simulink model "am_mod"  (R2023b)
settings: Solver=VariableStepAuto  StartTime=0.0  StopTime=0.1  RelTol=1e-3
values from neighbouring files (symbols this model uses):
  fc_mod_fm = 110e3    (= 110000)    [simulink_parametros.m]
  fc_test_mod_am = 10*fm_test_mod_am    (= 10000)    [simulink_parametros.m]
  fm_test_mod_am = 1000    [simulink_parametros.m]
  ts_test_mod_am = 1/fs_test_mod_am    (= 1e-05)    [simulink_parametros.m]
undefined symbols (not defined in the file or in its folder): BE, ode23tb, trap
libraries: rfmathmodels2 x1
settings Model: Creator=RomaW11  LastModifiedBy=RomaW11

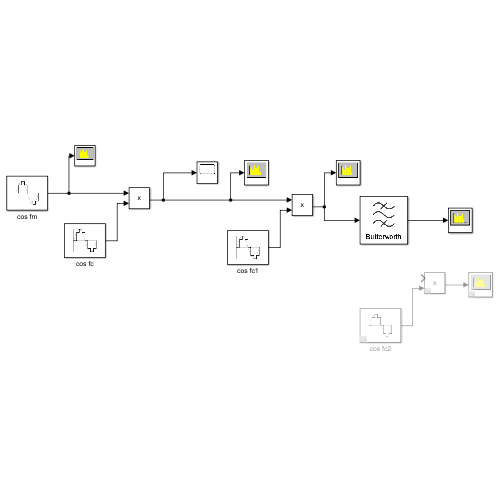
[thumbnail: Simulink's stored preview of the top-level diagram]
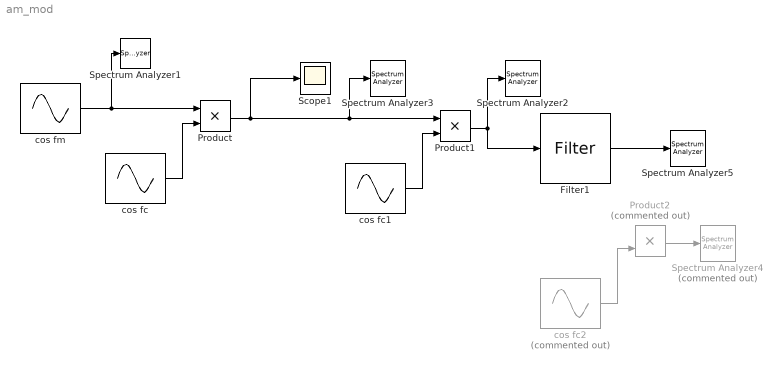
== system am_mod ==
  Filter1 : rfmathmodels2/Filter  DesignMethod=Butterworth  ResponseType=Bandpass  UseFilterOrder=on  FilterOrder=3  PassFreq_lp=1e9  PassFreq_hp=2000000000  PassFreq_bp=[15e3 25e3]  PassFreq_bs=[1000000000 4000000000]  PassAtten=10*log10(2)  StopFreq_lp=2000000000  StopFreq_hp=1000000000  StopFreq_bp=[1500000000 3500000000]  StopFreq_bs=[2100000000 2900000000]  StopAtten=40  CarrierFrequency=20e3  SignalBandwidth=10000000  SimulateUsing=Interpreted execution  ModelingDomain=Time domain (Fixed step)  SolverFixedStep=NDF2  SolverODE=ode23tb (trap+BE)  PoleFitting=Share all poles  RationalArguments={ 'Tolerance', -40, 'TendsToZero', false, 'MaxPoles', 48, 'Qlimit', inf }  LengthFIR=128  PlotType1=S21  Plot1Units=Magnitude (dB)  Plot1ArgumentsImpulse=[1e-11 1e4]  Plot1ArgumentsStep=[1e-11 1e4 1e-10]  PlotType2=None  Plot2Units=Magnitude (dB)  Plot2ArgumentsImpulse=[1e-11 1e4]  Plot2ArgumentsStep=[1e-11 1e4 1e-10]  FrequencyPoints=logspace(8,10,2001)  XaxisScale=Linear  YaxisScale=Linear
  Product : Product
  Product1 : Product
  Product2 : Product  Commented=on
  Scope1 : Scope
  Spectrum Analyzer1 : SpectrumAnalyzer  WindowPosition=[7.000000,-1079.000000,1920.000000,1057.000000,]  ScopeFrameLocation=window  SampleRate=44.1e3  StartFrequency=20  StopFrequency=20e3  YLimits=[-53.06122828,27.41733441]
      settings: OpenAtSimulationStart=off
  Spectrum Analyzer2 : SpectrumAnalyzer  WindowPosition=[7.000000,-1079.000000,1920.000000,1057.000000,]  ScopeFrameLocation=window  SampleRate=44.1e3  StartFrequency=20  StopFrequency=20e3  YLimits=[-52.30886083,20.64603656]  SelectedToolstripTab=spectrumAnalyzerToolstrip.estimationTab
      settings: OpenAtSimulationStart=off
  Spectrum Analyzer3 : SpectrumAnalyzer  WindowPosition=[1.000000,1.000000,1920.000000,1057.000000,]  ScopeFrameLocation=window  SampleRate=44.1e3  StartFrequency=20  StopFrequency=20e3  YLimits=[-52.32816931,20.81980716]
      settings: OpenAtSimulationStart=off
  Spectrum Analyzer4 : SpectrumAnalyzer  Commented=on  WindowPosition=[1.000000,1.000000,1920.000000,1057.000000,]  ScopeFrameLocation=window  SampleRate=44.1e3  StartFrequency=20  StopFrequency=20e3  YLimits=[-51.57709306,14.06031154]  SelectedToolstripTab=spectrumAnalyzerToolstrip.estimationTab
      settings: OpenAtSimulationStart=off
  Spectrum Analyzer5 : SpectrumAnalyzer  WindowPosition=[7.000000,-1079.000000,1920.000000,1057.000000,]  ScopeFrameLocation=window  SampleRate=44.1e3  StartFrequency=20  StopFrequency=20e3  YLimits=[-51.57709306,14.06031154]  SelectedToolstripTab=spectrumAnalyzerToolstrip.estimationTab
      settings: OpenAtSimulationStart=off
  cos fc : Sin  Frequency=2*pi*fc_test_mod_am  Phase=pi/2  SampleTime=ts_test_mod_am
  cos fc1 : Sin  Frequency=2*pi*fc_mod_fm  Phase=pi/2  SampleTime=ts_test_mod_am
  cos fc2 : Sin  Commented=on  Frequency=2*pi*fc_mod_fm*2  Phase=pi/2  SampleTime=ts_test_mod_am
  cos fm : Sin  Frequency=2*pi*fm_test_mod_am  Phase=pi/2  SampleTime=ts_test_mod_am
  wires:
  cos fc/1 -> Product/2
  cos fm/1 -> Spectrum Analyzer1/1, Product/1
  Product/1 -> Scope1/1, Product1/1, Spectrum Analyzer3/1
  cos fc1/1 -> Product1/2
  cos fc2/1 -> Product2/2
  Product2/1 -> Spectrum Analyzer4/1
  Product1/1 -> Filter1/1, Spectrum Analyzer2/1
  Filter1/1 -> Spectrum Analyzer5/1
